simulink subsystem "Piero_Modelo"  (R2023b)
settings: Solver=VariableStepAuto  StartTime=0.0  StopTime=10.0  RelTol=1e-3
settings Model: Creator=Enrique  LastModifiedBy=Enrique

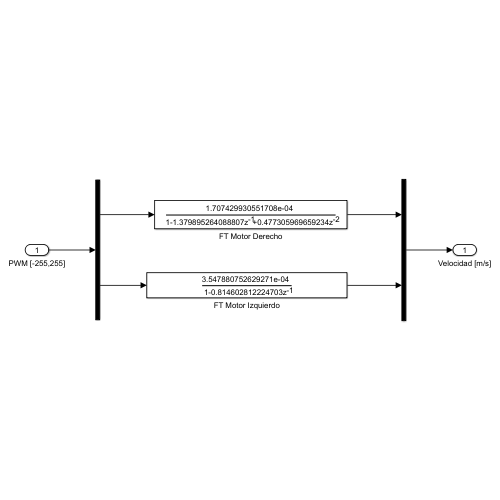
[thumbnail: Simulink's stored preview of the top-level diagram]
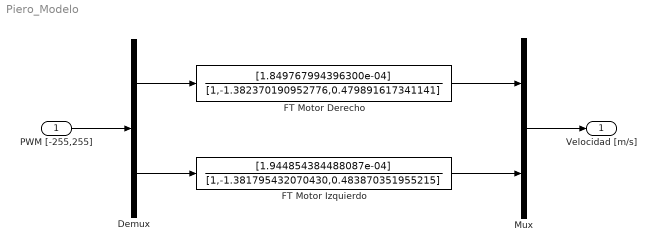
== system Piero_Modelo ==
  PWM [-255,255] : Inport
  Demux : Demux  Outputs=2
  FT Motor Derecho : DiscreteFilter  Numerator=[1.849767994396300e-04]  Denominator=[1,-1.382370190952776,0.479891617341141]
  FT Motor Izquierdo : DiscreteFilter  Numerator=[1.944854384488087e-04]  Denominator=[1,-1.381795432070430,0.483870351955215]
  Mux : Mux  Inputs=2
  Velocidad [m/s] : Outport
  wires:
  PWM [-255,255]/1 -> Demux/1
  Demux/1 -> FT Motor Derecho/1
  Demux/2 -> FT Motor Izquierdo/1
  Mux/1 -> Velocidad [m/s]/1
  FT Motor Derecho/1 -> Mux/1
  FT Motor Izquierdo/1 -> Mux/2
